simulink model "bouncing_ball"  (Simulink 7.4)
settings: Solver=ode45  StartTime=0.0  StopTime=10  RelTol=1e-3
libraries: vrlib x2
settings Model: Creator=smahapat  LastModifiedBy=jghidell

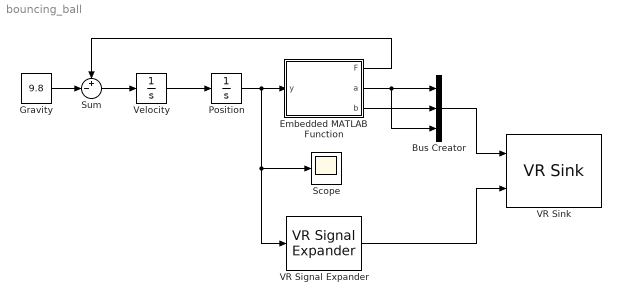
== system bouncing_ball ==
  Bus Creator : BusCreator  Inputs=3
  Embedded MATLAB Function : Stateflow chart
  Gravity : Constant  Value=9.8  OutDataType=fixdt(1, 16)  OutScaling=2^0
  Position : Integrator  InitialCondition=20
  Scope : Scope
      settings: YMin=0  YMax=22.5
  Sum : Sum  Inputs=+-|  OutDataType=fixdt(1, 16)  OutScaling=2^0
  VR Signal Expander : vrlib/VR Signal Expander  SystemSampleTime=-1  outwidth=3  outidx=[2]
  VR Sink : vrlib/VR Sink  InstantiateOnLoad=on  SampleTime=0.01  ViewEnable=on  RemoteChange=off  RemoteView=on  FieldsWritten=Ball.scale.3.1.double#Ball.translation.3.1.double  WorldFileName=bouncing_ball.wrl  AutoView=off  VideoDimensions=[]
  Velocity : Integrator
  wires:
  Velocity/1 -> Position/1
  Position/1 -> Embedded MATLAB Function/1(y), VR Signal Expander/1, Scope/1
  Sum/1 -> Velocity/1
  VR Signal Expander/1 -> VR Sink/2
  Bus Creator/1 -> VR Sink/1
  Embedded MATLAB Function/3(b) -> Bus Creator/2
  Embedded MATLAB Function/2(a) -> Bus Creator/1, Bus Creator/3
  Embedded MATLAB Function/1(F) -> Sum/1
  Gravity/1 -> Sum/2

== matlab function Embedded MATLAB Function ==
  data: F output double; a output double; b output double; y input double
function [F,a, b] = fcn(y)
%#eml

if y<1e-4
    y=1e-4;
end

if y<1.5
    f=500*(1.5-y);
    a=sqrt(1.5^3/y);
    b=y;
else
    f=0;
    a=1.5;
    b=1.5;
end
